simulink model "PositionControl"  (R2020b)
settings: Solver=ode3  StartTime=0.0  StopTime=100.0  FixedStep=Ts  RelTol=1e-3
values from neighbouring files (symbols this model uses):
  refx = 10*rand    [Ejercicio1.m]
  refy = 10*rand    [Ejercicio1.m]
undefined symbols (not defined in the file or in its folder): DiscIntNeverNeededParam
libraries: fuzblock x1, simulink x1
settings Model: Creator=patri  LastModifiedBy=Victor
settings DataIOCC: ReturnWorkspaceOutputs=off

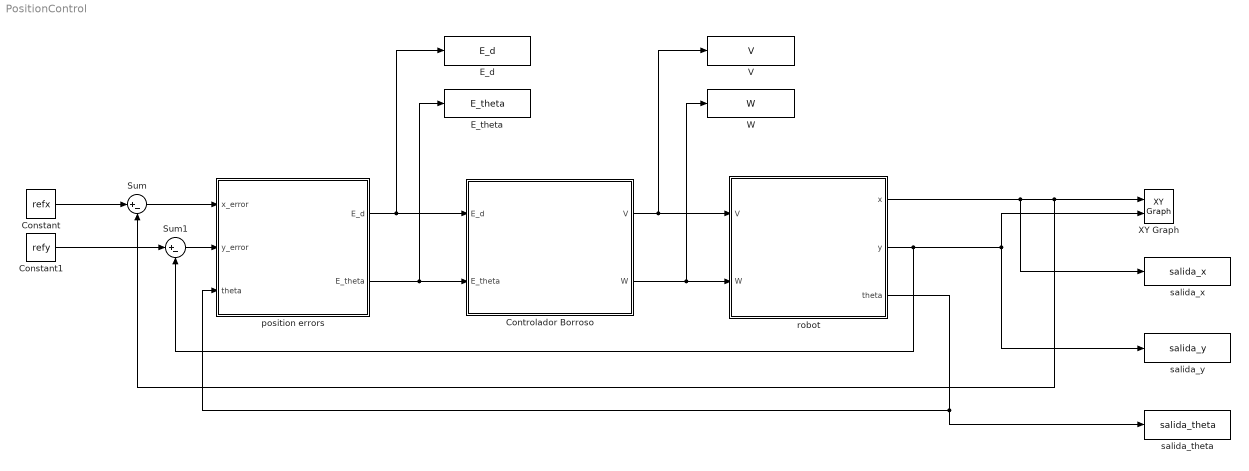
== system PositionControl ==
  Constant : Constant  Value=refx
  Constant1 : Constant  Value=refy
  Controlador Borroso : Subsystem
  E_d : ToWorkspace  VariableName=E_d  SaveFormat=Structure With Time  SampleTime=-1
  E_theta : ToWorkspace  VariableName=E_theta  SaveFormat=Structure With Time  SampleTime=-1
  Sum : Sum  Inputs=|+-
  Sum1 : Sum  Inputs=|+-
  V : ToWorkspace  VariableName=V  SaveFormat=Structure With Time  SampleTime=-1
  W : ToWorkspace  VariableName=W  SaveFormat=Structure With Time  SampleTime=-1
  XY Graph : simulink/Sinks/XY Graph  xmin=-20  xmax=20  ymin=-20  ymax=20  st=-1
  position errors : Subsystem
  robot : Subsystem
  salida_theta : ToWorkspace  VariableName=salida_theta  SaveFormat=Structure With Time  SampleTime=-1
  salida_x : ToWorkspace  VariableName=salida_x  SaveFormat=Structure With Time  SampleTime=-1
  salida_y : ToWorkspace  VariableName=salida_y  SaveFormat=Structure With Time  SampleTime=-1
  wires:
  Controlador Borroso/1(V) -> robot/1(V), V/1
  position errors/1(E_d) -> E_d/1, Controlador Borroso/1(E_d)
  robot/1(x) -> salida_x/1, Sum/2, XY Graph/1
  Controlador Borroso/2(W) -> robot/2(W), W/1
  robot/2(y) -> Sum1/2, salida_y/1, XY Graph/2
  robot/3(theta) -> salida_theta/1, position errors/3(theta)
  position errors/2(E_theta) -> E_theta/1, Controlador Borroso/2(E_theta)
  Constant/1 -> Sum/1
  Constant1/1 -> Sum1/1
  Sum1/1 -> position errors/2(y_error)
  Sum/1 -> position errors/1(x_error)

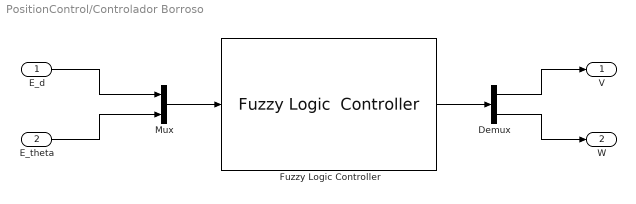
== system PositionControl/Controlador Borroso ==
  E_d : Inport
  E_theta : Inport  Port=2
  Demux : Demux  Outputs=2
  Fuzzy Logic Controller : fuzblock/Fuzzy Logic  Controller  FIS='ControlBorroso.fis'  OutputSampleNumber=101  DataType=double  FuzzifiedInputs=off  RuleFiringStrengths=off  RuleOutputs=off  AggregatedOutputs=off  SimulateUsing=Interpreted execution  OutOfRangeInputValueMessage=warning  NoRuleFiredMessage=warning  EmptyOutputFuzzySetMessage=warning
  Mux : Mux  Inputs=2
  V : Outport
  W : Outport  Port=2
  wires:
  Mux/1 -> Fuzzy Logic Controller/1
  E_theta/1 -> Mux/2
  Demux/1 -> V/1
  Fuzzy Logic Controller/1 -> Demux/1
  E_d/1 -> Mux/1
  Demux/2 -> W/1

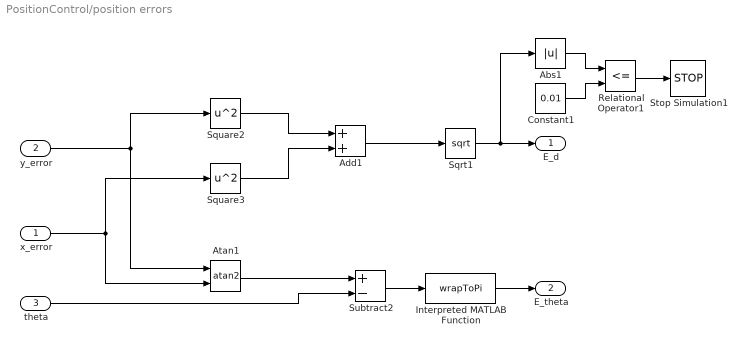
== system PositionControl/position errors ==
  x_error : Inport
  y_error : Inport  Port=2
  theta : Inport  Port=3
  Abs1 : Abs
  Add1 : Sum
  Atan1 : Trigonometry  Operator=atan2
  Constant1 : Constant  Value=0.01
  Interpreted MATLAB Function : MATLABFcn  MATLABFcn=wrapToPi
  Relational Operator1 : RelationalOperator  Operator=<=  OutDataTypeStr=boolean  RndMeth=Simplest
  Sqrt1 : Sqrt  SaturateOnIntegerOverflow=on
  Square2 : Math  Operator=square  SignedPower=on  SaturateOnIntegerOverflow=on
  Square3 : Math  Operator=square  SignedPower=on  SaturateOnIntegerOverflow=on
  Stop Simulation1 : Stop
  Subtract2 : Sum  Inputs=+-  OutMin=[-3.14]  OutMax=[3.14]
  E_d : Outport  VectorParamsAs1DForOutWhenUnconnected=off
  E_theta : Outport  Port=2  OutMin=[-pi]  OutMax=[pi]  VectorParamsAs1DForOutWhenUnconnected=off
  wires:
  Subtract2/1 -> Interpreted MATLAB Function/1
  Relational Operator1/1 -> Stop Simulation1/1
  Atan1/1 -> Subtract2/1
  x_error/1 -> Atan1/2, Square3/1
  Constant1/1 -> Relational Operator1/2
  Interpreted MATLAB Function/1 -> E_theta/1
  Abs1/1 -> Relational Operator1/1
  Square3/1 -> Add1/2
  Sqrt1/1 -> Abs1/1, E_d/1
  Square2/1 -> Add1/1
  Add1/1 -> Sqrt1/1
  theta/1 -> Subtract2/2
  y_error/1 -> Atan1/1, Square2/1

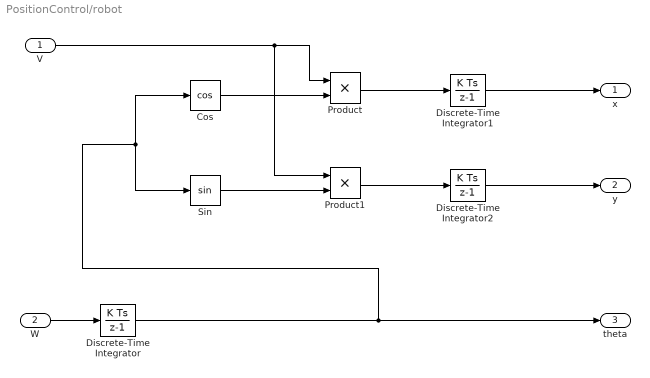
== system PositionControl/robot ==
  V : Inport
  W : Inport  Port=2
  Cos : Trigonometry  Operator=cos
  Discrete-Time Integrator : DiscreteIntegrator  SampleTime=-1  ICPrevOutput=DiscIntNeverNeededParam  ICPrevScaledInput=DiscIntNeverNeededParam
  Discrete-Time Integrator1 : DiscreteIntegrator  SampleTime=-1  ICPrevOutput=DiscIntNeverNeededParam  ICPrevScaledInput=DiscIntNeverNeededParam
  Discrete-Time Integrator2 : DiscreteIntegrator  SampleTime=-1  ICPrevOutput=DiscIntNeverNeededParam  ICPrevScaledInput=DiscIntNeverNeededParam
  Product : Product
  Product1 : Product
  Sin : Trigonometry
  x : Outport  VectorParamsAs1DForOutWhenUnconnected=off
  y : Outport  Port=2  VectorParamsAs1DForOutWhenUnconnected=off
  theta : Outport  Port=3  VectorParamsAs1DForOutWhenUnconnected=off
  wires:
  Discrete-Time Integrator2/1 -> y/1
  W/1 -> Discrete-Time Integrator/1
  Discrete-Time Integrator1/1 -> x/1
  Discrete-Time Integrator/1 -> theta/1, Sin/1, Cos/1
  Product1/1 -> Discrete-Time Integrator2/1
  Sin/1 -> Product1/2
  V/1 -> Product1/1, Product/1
  Product/1 -> Discrete-Time Integrator1/1
  Cos/1 -> Product/2
